simulink model "impulse_ex_discrete"  (R2024a)
settings: Solver=ode5  StartTime=0.0  StopTime=6  FixedStep=0.001  RelTol=1e-6  AbsTol=1e-6
undefined symbols (not defined in the file or in its folder): sys
settings Model: DataDictionary=impulseDD.sldd  Creator=grouleau  LastModifiedBy=grouleau

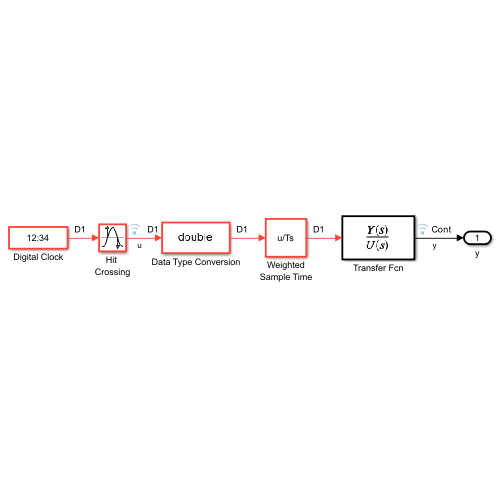
[thumbnail: Simulink's stored preview of the top-level diagram]
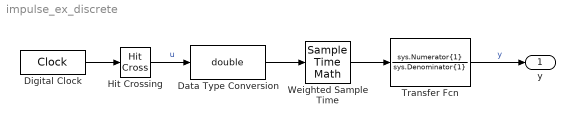
== system impulse_ex_discrete ==
  Data Type Conversion : DataTypeConversion  OutDataTypeStr=double  SaturateOnIntegerOverflow=off  RndMeth=Floor
  Digital Clock : DigitalClock  SampleTime=0.001
  Hit Crossing : HitCross  HitCrossingOffset=1
  Transfer Fcn : TransferFcn  Numerator=sys.Numerator{1}  Denominator=sys.Denominator{1}
  Weighted Sample Time : SampleTimeMath  TsampMathOp=/
  y : Outport
  wires:
  Transfer Fcn/1 -> y/1  "y"
  Hit Crossing/1 -> Data Type Conversion/1  "u"
  Digital Clock/1 -> Hit Crossing/1
  Weighted Sample Time/1 -> Transfer Fcn/1
  Data Type Conversion/1 -> Weighted Sample Time/1
